simulink model "System_composer__model_pre_alpha_V2"  (R2022b)
settings: Solver=VariableStepAuto  StartTime=0.0  StopTime=10.0  RelTol=1e-3
(part 1 of 3)
settings Model: Creator=user  LastModifiedBy=Sunil Kumar

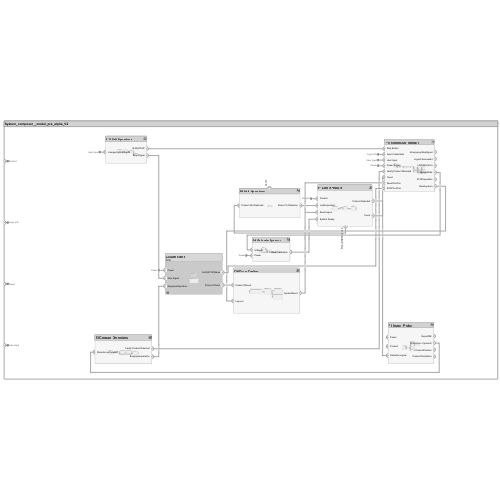
[thumbnail: Simulink's stored preview of the top-level diagram]
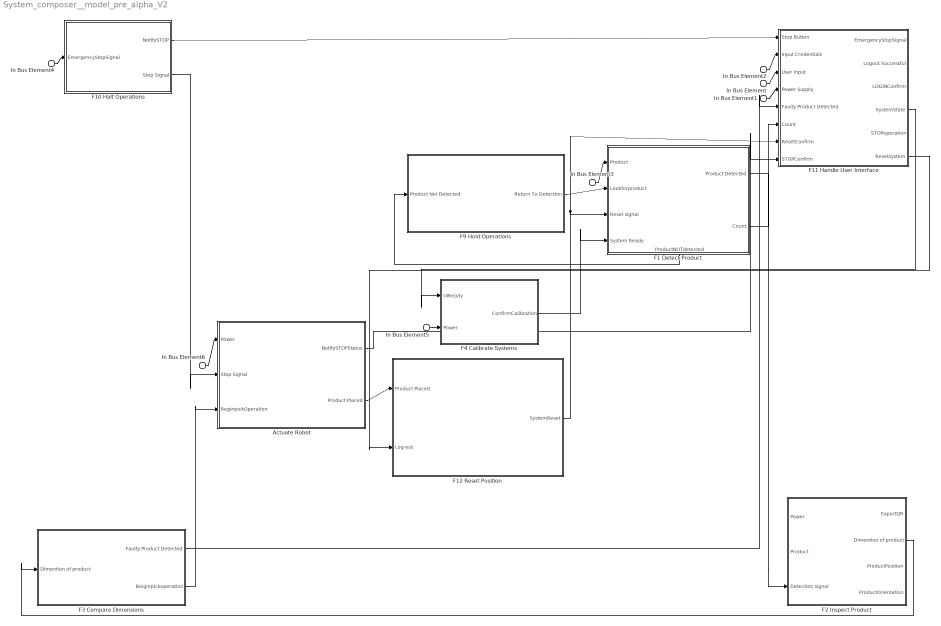
== system System_composer__model_pre_alpha_V2 ==
  In Bus Element3 : Inport  PortName=Product
  In Bus Element2 : Inport  Port=2  PortName=Login info
  In Bus Element1 : Inport  Port=3  PortName=Power
  In Bus Element6 : Inport  Port=3  PortName=Power
  In Bus Element5 : Inport  Port=3  PortName=Power
  In Bus Element : Inport  Port=4  PortName=User Input
  In Bus Element4 : Inport  Port=4  PortName=User Input
  Actuate Robot : Subsystem  Variant=on  VariantControlMode=label  LabelModeActiveChoice=false
      settings: PortSchema="{\"entries\":[{\"content\":{\"headerSize\":38,\"margin\":15,\"minimumSpacing\":25,\"sides\":[{\"content\":{\"connectorIds\":[\"In1\",\"In2\",\"In3\"]},\"type\":\"ConnectorPlacement.EquallySpacedRectSide\",\"uuid\":\"801652fd-f6d1-4274-af0e-cb86f9305aea\"},{\"content\":{\"connectorIds\":[\"Out1\",\"Out2\"],\"side\":\"RIGHT\"},\"type\":\"ConnectorPlacement.EquallySpacedRectSide\",\"uuid\":\"95203280-2c96-4067-b57a-d6395a07757b\"},{\"content\":{\"connectorIds\":[],\"side\":\"TOP\"},\"type\":\"ConnectorPlacement.EquallySpacedRectSide\",\"uuid\":\"56d65509-64de-4fc3-ae90-5c873f468874\"}]},\"type\":\"ConnectorPlacement.EquallySpacedConnector\",\"uuid\":\"1a0d29b8-31f4-46a4-bc3c-cb1d4cb15c15\"}],\"packageUris\":[\"http://schema.mathworks.com/mf0/Connector/R2020b\"],\"version\":\"1.0\"}"
  F1 Detect Product : Subsystem
      settings: PortSchema="{\"entries\":[{\"content\":{\"headerSize\":26,\"margin\":15,\"minimumSpacing\":25,\"sides\":[{\"content\":{\"connectorIds\":[\"In1\",\"In2\",\"In3\",\"In4\"]},\"type\":\"ConnectorPlacement.EquallySpacedRectSide\",\"uuid\":\"0eb90d47-70e1-4803-9acf-c665eca2c33b\"},{\"content\":{\"connectorIds\":[\"Out2\",\"Out3\"],\"side\":\"RIGHT\"},\"type\":\"ConnectorPlacement.EquallySpacedRectSide\",\"uuid\":\"4ca2a7b5-05ae-49c5-bdeb-54cebcfbfa14\"},{\"content\":{\"connectorIds\":[],\"side\":\"TOP\"},\"type\":\"ConnectorPlacement.EquallySpacedRectSide\",\"uuid\":\"0ca0afdf-f9df-4611-9068-250b443486a2\"},{\"content\":{\"connectorIds\":[\"Out1\"],\"side\":\"BOTTOM\"},\"type\":\"ConnectorPlacement.EquallySpacedRectSide\",\"uuid\":\"bd2a3fb3-3c9c-4a9d-a87c-821984a35fa0\"}]},\"type\":\"ConnectorPlacement.EquallySpacedConnector\",\"uuid\":\"958f48af-2ef9-4d0f-b00d-a4686f354a93\"}],\"packageUris\":[\"http://schema.mathworks.com/mf0/Connector/R2020b\"],\"version\":\"1.0\"}"
  F10 Halt Operations : Subsystem
      settings: PortSchema="{\"entries\":[{\"content\":{\"headerSize\":26,\"margin\":15,\"minimumSpacing\":25,\"sides\":[{\"content\":{\"connectorIds\":[\"In1\"]},\"type\":\"ConnectorPlacement.EquallySpacedRectSide\",\"uuid\":\"0eb90d47-70e1-4803-9acf-c665eca2c33b\"},{\"content\":{\"connectorIds\":[\"Out1\",\"Out2\"],\"side\":\"RIGHT\"},\"type\":\"ConnectorPlacement.EquallySpacedRectSide\",\"uuid\":\"4ca2a7b5-05ae-49c5-bdeb-54cebcfbfa14\"},{\"content\":{\"connectorIds\":[],\"side\":\"TOP\"},\"type\":\"ConnectorPlacement.EquallySpacedRectSide\",\"uuid\":\"0ca0afdf-f9df-4611-9068-250b443486a2\"}]},\"type\":\"ConnectorPlacement.EquallySpacedConnector\",\"uuid\":\"958f48af-2ef9-4d0f-b00d-a4686f354a93\"}],\"packageUris\":[\"http://schema.mathworks.com/mf0/Connector/R2020b\"],\"version\":\"1.0\"}"
  F11 Handle User Interface : Subsystem
      settings: PortSchema="{\"entries\":[{\"content\":{\"headerSize\":26,\"margin\":15,\"minimumSpacing\":25,\"sides\":[{\"content\":{\"connectorIds\":[\"In1\",\"In2\",\"In3\",\"In4\",\"In5\",\"In6\",\"In7\",\"In8\"]},\"type\":\"ConnectorPlacement.EquallySpacedRectSide\",\"uuid\":\"0eb90d47-70e1-4803-9acf-c665eca2c33b\"},{\"content\":{\"connectorIds\":[\"Out1\",\"Out2\",\"Out3\",\"Out5\",\"Out6\",\"Out4\"],\"side\":\"RIGHT\"},\"type\":\"ConnectorPlacement.EquallySpacedRectSide\",\"uuid\":\"4ca2a7b5-05ae-49c5-bdeb-54cebcfbfa14\"},{\"content\":{\"connectorIds\":[],\"side\":\"TOP\"},\"type\":\"ConnectorPlacement.EquallySpacedRectSide\",\"uuid\":\"0ca0afdf-f9df-4611-9068-250b443486a2\"}]},\"type\":\"ConnectorPlacement.EquallySpacedConnector\",\"uuid\":\"958f48af-2ef9-4d0f-b00d-a4686f354a93\"}],\"packageUris\":[\"http://schema.mathworks.com/mf0/Connector/R2020b\"],\"version\":\"1.0\"}"
  F12 Reset Position : Subsystem
      settings: PortSchema="{\"entries\":[{\"content\":{\"headerSize\":26,\"margin\":15,\"minimumSpacing\":25,\"sides\":[{\"content\":{\"connectorIds\":[\"In1\",\"In2\"]},\"type\":\"ConnectorPlacement.EquallySpacedRectSide\",\"uuid\":\"1c117138-a6d4-4ec0-b7b8-6d1428745998\"},{\"content\":{\"connectorIds\":[\"Out1\"],\"side\":\"RIGHT\"},\"type\":\"ConnectorPlacement.EquallySpacedRectSide\",\"uuid\":\"426d6ceb-18a6-42d8-9bd7-8fe69cb751f0\"},{\"content\":{\"connectorIds\":[],\"side\":\"TOP\"},\"type\":\"ConnectorPlacement.EquallySpacedRectSide\",\"uuid\":\"23012487-78cd-45b9-9306-44393710ac2e\"}]},\"type\":\"ConnectorPlacement.EquallySpacedConnector\",\"uuid\":\"f4468a7a-13e2-43af-b621-864ee5d109de\"}],\"packageUris\":[\"http://schema.mathworks.com/mf0/Connector/R2020b\"],\"version\":\"1.0\"}"
  F2 Inspect Product : Subsystem
      settings: PortSchema="{\"entries\":[{\"content\":{\"headerSize\":26,\"margin\":15,\"minimumSpacing\":25,\"sides\":[{\"content\":{\"connectorIds\":[\"In1\",\"In2\",\"In3\"]},\"type\":\"ConnectorPlacement.EquallySpacedRectSide\",\"uuid\":\"0eb90d47-70e1-4803-9acf-c665eca2c33b\"},{\"content\":{\"connectorIds\":[\"Out1\",\"Out2\",\"Out3\",\"Out4\"],\"side\":\"RIGHT\"},\"type\":\"ConnectorPlacement.EquallySpacedRectSide\",\"uuid\":\"4ca2a7b5-05ae-49c5-bdeb-54cebcfbfa14\"},{\"content\":{\"connectorIds\":[],\"side\":\"TOP\"},\"type\":\"ConnectorPlacement.EquallySpacedRectSide\",\"uuid\":\"0ca0afdf-f9df-4611-9068-250b443486a2\"}]},\"type\":\"ConnectorPlacement.EquallySpacedConnector\",\"uuid\":\"958f48af-2ef9-4d0f-b00d-a4686f354a93\"}],\"packageUris\":[\"http://schema.mathworks.com/mf0/Connector/R2020b\"],\"version\":\"1.0\"}"
  F3 Compare Dimensions : Subsystem
      settings: PortSchema="{\"entries\":[{\"content\":{\"headerSize\":26,\"margin\":15,\"minimumSpacing\":25,\"sides\":[{\"content\":{\"connectorIds\":[\"In1\"]},\"type\":\"ConnectorPlacement.EquallySpacedRectSide\",\"uuid\":\"0eb90d47-70e1-4803-9acf-c665eca2c33b\"},{\"content\":{\"connectorIds\":[\"Out1\",\"Out2\"],\"side\":\"RIGHT\"},\"type\":\"ConnectorPlacement.EquallySpacedRectSide\",\"uuid\":\"4ca2a7b5-05ae-49c5-bdeb-54cebcfbfa14\"},{\"content\":{\"connectorIds\":[],\"side\":\"TOP\"},\"type\":\"ConnectorPlacement.EquallySpacedRectSide\",\"uuid\":\"0ca0afdf-f9df-4611-9068-250b443486a2\"}]},\"type\":\"ConnectorPlacement.EquallySpacedConnector\",\"uuid\":\"958f48af-2ef9-4d0f-b00d-a4686f354a93\"}],\"packageUris\":[\"http://schema.mathworks.com/mf0/Connector/R2020b\"],\"version\":\"1.0\"}"
  "F4 Calibrate Systems " : Subsystem
      settings: PortSchema="{\"entries\":[{\"content\":{\"headerSize\":26,\"margin\":15,\"minimumSpacing\":25,\"sides\":[{\"content\":{\"connectorIds\":[\"In1\",\"In2\"]},\"type\":\"ConnectorPlacement.EquallySpacedRectSide\",\"uuid\":\"0eb90d47-70e1-4803-9acf-c665eca2c33b\"},{\"content\":{\"connectorIds\":[\"Out1\"],\"side\":\"RIGHT\"},\"type\":\"ConnectorPlacement.EquallySpacedRectSide\",\"uuid\":\"4ca2a7b5-05ae-49c5-bdeb-54cebcfbfa14\"},{\"content\":{\"connectorIds\":[],\"side\":\"TOP\"},\"type\":\"ConnectorPlacement.EquallySpacedRectSide\",\"uuid\":\"0ca0afdf-f9df-4611-9068-250b443486a2\"}]},\"type\":\"ConnectorPlacement.EquallySpacedConnector\",\"uuid\":\"958f48af-2ef9-4d0f-b00d-a4686f354a93\"}],\"packageUris\":[\"http://schema.mathworks.com/mf0/Connector/R2020b\"],\"version\":\"1.0\"}"
  F9 Hold Operations : Subsystem
      settings: PortSchema="{\"entries\":[{\"content\":{\"headerSize\":26,\"margin\":15,\"minimumSpacing\":25,\"sides\":[{\"content\":{\"connectorIds\":[\"In1\"]},\"type\":\"ConnectorPlacement.EquallySpacedRectSide\",\"uuid\":\"0eb90d47-70e1-4803-9acf-c665eca2c33b\"},{\"content\":{\"connectorIds\":[\"Out1\"],\"side\":\"RIGHT\"},\"type\":\"ConnectorPlacement.EquallySpacedRectSide\",\"uuid\":\"4ca2a7b5-05ae-49c5-bdeb-54cebcfbfa14\"},{\"content\":{\"connectorIds\":[\"LConn1\"],\"side\":\"TOP\"},\"type\":\"ConnectorPlacement.EquallySpacedRectSide\",\"uuid\":\"0ca0afdf-f9df-4611-9068-250b443486a2\"}]},\"type\":\"ConnectorPlacement.EquallySpacedConnector\",\"uuid\":\"958f48af-2ef9-4d0f-b00d-a4686f354a93\"}],\"packageUris\":[\"http://schema.mathworks.com/mf0/Connector/R2020b\"],\"version\":\"1.0\"}"
  wires:
  In Bus Element4/1 -> F10 Halt Operations/1(EmergencyStopSignal)
  F10 Halt Operations/1(NotifySTOP) -> F11 Handle User Interface/1(Stop Button)
  F3 Compare Dimensions/2(Beiginpickoperation) -> Actuate Robot/3(BeginpickOperation)
  F3 Compare Dimensions/1(Faulty Product Detected) -> F11 Handle User Interface/5(Faulty Product Detected)
  F1 Detect Product/2(Product Detected) -> F2 Inspect Product/3(Detection signal)
  F10 Halt Operations/2(Stop Signal) -> Actuate Robot/2(Stop Signal)
  Actuate Robot/2(Product Placed) -> F12 Reset Position/1(Product Placed)
  In Bus Element6/1 -> Actuate Robot/1(Power)
  F11 Handle User Interface/4(Resetsystem) -> F12 Reset Position/2(Log-out)
  Actuate Robot/1(NotifySTOPStatus) -> F11 Handle User Interface/8(STOPConfirm)
  In Bus Element5/1 -> "F4 Calibrate Systems "/2(Power)
  In Bus Element3/1 -> F1 Detect Product/1(Product)
  F9 Hold Operations/1(Return To Detection) -> F1 Detect Product/2(Lookforproduct)
  "F4 Calibrate Systems "/1(ConfirmCalibration) -> F1 Detect Product/4(System Ready)
  F12 Reset Position/1(SystemReset) -> F11 Handle User Interface/7(ResetConfirm), F1 Detect Product/3(Reset signal)
  F1 Detect Product/3(Count) -> F11 Handle User Interface/6(Count)
  F1 Detect Product/1(ProductNOTdetected) -> F9 Hold Operations/1(Product Not Detected)
  In Bus Element2/1 -> F11 Handle User Interface/2(Input Credentials)
  In Bus Element/1 -> F11 Handle User Interface/3(User Input)
  In Bus Element1/1 -> F11 Handle User Interface/4(Power Supply)
  F11 Handle User Interface/5(SystemState) -> "F4 Calibrate Systems "/1(UIReady)
  F2 Inspect Product/2(Dimention of product) -> F3 Compare Dimensions/1(Dimention of product)

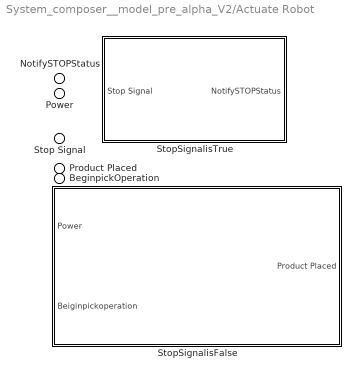
== system System_composer__model_pre_alpha_V2/Actuate Robot ==
  Power : Inport
  Stop Signal : Inport  Port=2
  BeginpickOperation : Inport  Port=3
  StopSignalisFalse : Subsystem  VariantControl=false
      settings: PortSchema="{\"entries\":[{\"content\":{\"headerSize\":26,\"margin\":15,\"minimumSpacing\":25,\"sides\":[{\"content\":{\"connectorIds\":[\"In1\",\"In2\"]},\"type\":\"ConnectorPlacement.EquallySpacedRectSide\",\"uuid\":\"48af5bc1-3520-4798-93f0-e999f4a2b359\"},{\"content\":{\"connectorIds\":[\"Out1\"],\"side\":\"RIGHT\"},\"type\":\"ConnectorPlacement.EquallySpacedRectSide\",\"uuid\":\"b080505c-f688-49a6-aa0b-291a70fb9613\"},{\"content\":{\"connectorIds\":[],\"side\":\"TOP\"},\"type\":\"ConnectorPlacement.EquallySpacedRectSide\",\"uuid\":\"3b22725c-7b13-4de8-bd12-2bd6e95657e0\"}]},\"type\":\"ConnectorPlacement.EquallySpacedConnector\",\"uuid\":\"97afaf3e-8205-465e-91b8-6c9d28738099\"}],\"packageUris\":[\"http://schema.mathworks.com/mf0/Connector/R2020b\"],\"version\":\"1.0\"}"
  StopSignalisTrue : Subsystem  VariantControl=true
      settings: PortSchema="{\"entries\":[{\"content\":{\"headerSize\":26,\"margin\":15,\"minimumSpacing\":25,\"sides\":[{\"content\":{\"connectorIds\":[\"In1\"]},\"type\":\"ConnectorPlacement.EquallySpacedRectSide\",\"uuid\":\"48af5bc1-3520-4798-93f0-e999f4a2b359\"},{\"content\":{\"connectorIds\":[\"Out1\"],\"side\":\"RIGHT\"},\"type\":\"ConnectorPlacement.EquallySpacedRectSide\",\"uuid\":\"b080505c-f688-49a6-aa0b-291a70fb9613\"},{\"content\":{\"connectorIds\":[],\"side\":\"TOP\"},\"type\":\"ConnectorPlacement.EquallySpacedRectSide\",\"uuid\":\"3b22725c-7b13-4de8-bd12-2bd6e95657e0\"}]},\"type\":\"ConnectorPlacement.EquallySpacedConnector\",\"uuid\":\"97afaf3e-8205-465e-91b8-6c9d28738099\"}],\"packageUris\":[\"http://schema.mathworks.com/mf0/Connector/R2020b\"],\"version\":\"1.0\"}"
  NotifySTOPStatus : Outport
  Product Placed : Outport  Port=2

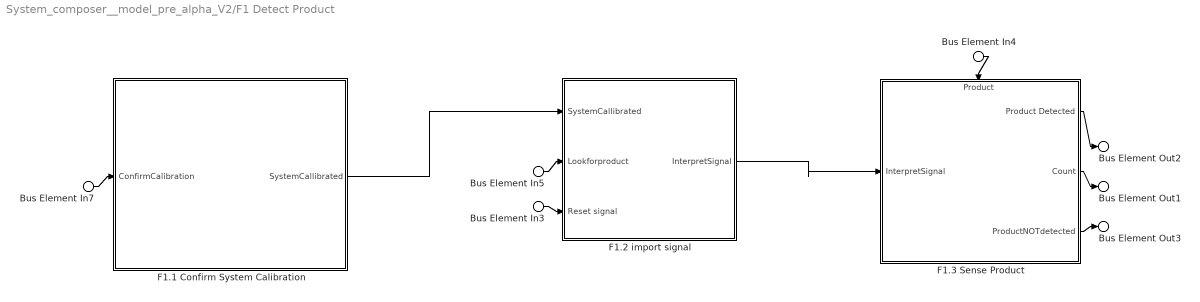
== system System_composer__model_pre_alpha_V2/F1 Detect Product ==
  Bus Element In4 : Inport  PortName=Product
  Bus Element In5 : Inport  Port=2  PortName=Lookforproduct
  Bus Element In3 : Inport  Port=3  PortName=Reset signal
  Bus Element In7 : Inport  Port=4  PortName=System Ready
  F1.1 Confirm System Calibration : Subsystem
      settings: PortSchema="{\"entries\":[{\"content\":{\"headerSize\":26,\"margin\":15,\"minimumSpacing\":25,\"sides\":[{\"content\":{\"connectorIds\":[\"In1\"]},\"type\":\"ConnectorPlacement.EquallySpacedRectSide\",\"uuid\":\"ae240f5f-39ed-41a3-b9a8-bf2f33b986be\"},{\"content\":{\"connectorIds\":[\"Out1\"],\"side\":\"RIGHT\"},\"type\":\"ConnectorPlacement.EquallySpacedRectSide\",\"uuid\":\"44ba199a-fd12-4621-8565-f3f1adedec4a\"},{\"content\":{\"connectorIds\":[],\"side\":\"TOP\"},\"type\":\"ConnectorPlacement.EquallySpacedRectSide\",\"uuid\":\"41d301d8-0f91-4ed1-b07b-750dd04e1ae2\"}]},\"type\":\"ConnectorPlacement.EquallySpacedConnector\",\"uuid\":\"8d081691-644b-416f-87ea-d7e0a52b2ce6\"}],\"packageUris\":[\"http://schema.mathworks.com/mf0/Connector/R2020b\"],\"version\":\"1.0\"}"
  F1.2 import signal : Subsystem
      settings: PortSchema="{\"entries\":[{\"content\":{\"headerSize\":26,\"margin\":15,\"minimumSpacing\":25,\"sides\":[{\"content\":{\"connectorIds\":[\"In1\",\"In2\",\"In3\"]},\"type\":\"ConnectorPlacement.EquallySpacedRectSide\",\"uuid\":\"ee97644e-c9ff-4946-8a58-fee1d557a4ad\"},{\"content\":{\"connectorIds\":[\"Out1\"],\"side\":\"RIGHT\"},\"type\":\"ConnectorPlacement.EquallySpacedRectSide\",\"uuid\":\"e20fd496-d0ba-45f7-949d-94f28912a261\"},{\"content\":{\"connectorIds\":[],\"side\":\"TOP\"},\"type\":\"ConnectorPlacement.EquallySpacedRectSide\",\"uuid\":\"6224eb33-55c0-4770-9979-a18202099dbf\"}]},\"type\":\"ConnectorPlacement.EquallySpacedConnector\",\"uuid\":\"f8ef62f6-ad53-4f25-bdc3-ef7ca131dedb\"}],\"packageUris\":[\"http://schema.mathworks.com/mf0/Connector/R2020b\"],\"version\":\"1.0\"}"
  F1.3 Sense Product : Subsystem
      settings: PortSchema="{\"entries\":[{\"content\":{\"headerSize\":26,\"margin\":15,\"minimumSpacing\":25,\"sides\":[{\"content\":{\"connectorIds\":[\"In2\"]},\"type\":\"ConnectorPlacement.EquallySpacedRectSide\",\"uuid\":\"ee97644e-c9ff-4946-8a58-fee1d557a4ad\"},{\"content\":{\"connectorIds\":[\"Out1\",\"Out2\",\"Out3\"],\"side\":\"RIGHT\"},\"type\":\"ConnectorPlacement.EquallySpacedRectSide\",\"uuid\":\"e20fd496-d0ba-45f7-949d-94f28912a261\"},{\"content\":{\"connectorIds\":[\"In1\"],\"side\":\"TOP\"},\"type\":\"ConnectorPlacement.EquallySpacedRectSide\",\"uuid\":\"6224eb33-55c0-4770-9979-a18202099dbf\"}]},\"type\":\"ConnectorPlacement.EquallySpacedConnector\",\"uuid\":\"f8ef62f6-ad53-4f25-bdc3-ef7ca131dedb\"}],\"packageUris\":[\"http://schema.mathworks.com/mf0/Connector/R2020b\"],\"version\":\"1.0\"}"
  Bus Element Out3 : Outport  PortName=ProductNOTdetected
  Bus Element Out2 : Outport  Port=2  PortName=Product Detected
  Bus Element Out1 : Outport  Port=3  PortName=Count
  wires:
  Bus Element In3/1 -> F1.2 import signal/3(Reset signal)
  F1.2 import signal/1(InterpretSignal) -> F1.3 Sense Product/2(InterpretSignal)
  Bus Element In4/1 -> F1.3 Sense Product/1(Product)
  F1.3 Sense Product/2(Count) -> Bus Element Out1/1
  F1.3 Sense Product/1(Product Detected) -> Bus Element Out2/1
  F1.3 Sense Product/3(ProductNOTdetected) -> Bus Element Out3/1
  Bus Element In5/1 -> F1.2 import signal/2(Lookforproduct)
  F1.1 Confirm System Calibration/1(SystemCallibrated) -> F1.2 import signal/1(SystemCallibrated)
  Bus Element In7/1 -> F1.1 Confirm System Calibration/1(ConfirmCalibration)

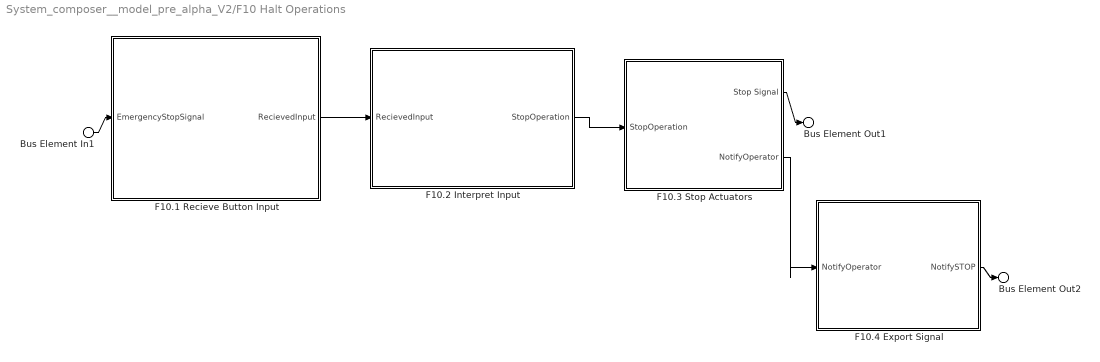
== system System_composer__model_pre_alpha_V2/F10 Halt Operations ==
  Bus Element In1 : Inport  PortName=EmergencyStopSignal
  F10.1 Recieve Button Input : Subsystem
      settings: PortSchema="{\"entries\":[{\"content\":{\"headerSize\":26,\"margin\":15,\"minimumSpacing\":25,\"sides\":[{\"content\":{\"connectorIds\":[\"In1\"]},\"type\":\"ConnectorPlacement.EquallySpacedRectSide\",\"uuid\":\"7013333b-bcb0-472a-8b4b-201a684e0f69\"},{\"content\":{\"connectorIds\":[\"Out1\"],\"side\":\"RIGHT\"},\"type\":\"ConnectorPlacement.EquallySpacedRectSide\",\"uuid\":\"4b4cc890-b976-4837-92a8-5b6c4ad3f659\"},{\"content\":{\"connectorIds\":[],\"side\":\"TOP\"},\"type\":\"ConnectorPlacement.EquallySpacedRectSide\",\"uuid\":\"d943cfaa-ae22-4a3b-a19a-c6fb5e90d8f6\"}]},\"type\":\"ConnectorPlacement.EquallySpacedConnector\",\"uuid\":\"02e5c76f-f132-4257-84b4-ea3020272a7a\"}],\"packageUris\":[\"http://schema.mathworks.com/mf0/Connector/R2020b\"],\"version\":\"1.0\"}"
  F10.2 Interpret Input : Subsystem
      settings: PortSchema="{\"entries\":[{\"content\":{\"headerSize\":26,\"margin\":15,\"minimumSpacing\":25,\"sides\":[{\"content\":{\"connectorIds\":[\"In1\"]},\"type\":\"ConnectorPlacement.EquallySpacedRectSide\",\"uuid\":\"7013333b-bcb0-472a-8b4b-201a684e0f69\"},{\"content\":{\"connectorIds\":[\"Out1\"],\"side\":\"RIGHT\"},\"type\":\"ConnectorPlacement.EquallySpacedRectSide\",\"uuid\":\"4b4cc890-b976-4837-92a8-5b6c4ad3f659\"},{\"content\":{\"connectorIds\":[],\"side\":\"TOP\"},\"type\":\"ConnectorPlacement.EquallySpacedRectSide\",\"uuid\":\"d943cfaa-ae22-4a3b-a19a-c6fb5e90d8f6\"}]},\"type\":\"ConnectorPlacement.EquallySpacedConnector\",\"uuid\":\"02e5c76f-f132-4257-84b4-ea3020272a7a\"}],\"packageUris\":[\"http://schema.mathworks.com/mf0/Connector/R2020b\"],\"version\":\"1.0\"}"
  F10.3 Stop Actuators : Subsystem
      settings: PortSchema="{\"entries\":[{\"content\":{\"headerSize\":26,\"margin\":15,\"minimumSpacing\":25,\"sides\":[{\"content\":{\"connectorIds\":[\"In1\"]},\"type\":\"ConnectorPlacement.EquallySpacedRectSide\",\"uuid\":\"7013333b-bcb0-472a-8b4b-201a684e0f69\"},{\"content\":{\"connectorIds\":[\"Out2\",\"Out1\"],\"side\":\"RIGHT\"},\"type\":\"ConnectorPlacement.EquallySpacedRectSide\",\"uuid\":\"4b4cc890-b976-4837-92a8-5b6c4ad3f659\"},{\"content\":{\"connectorIds\":[],\"side\":\"TOP\"},\"type\":\"ConnectorPlacement.EquallySpacedRectSide\",\"uuid\":\"d943cfaa-ae22-4a3b-a19a-c6fb5e90d8f6\"}]},\"type\":\"ConnectorPlacement.EquallySpacedConnector\",\"uuid\":\"02e5c76f-f132-4257-84b4-ea3020272a7a\"}],\"packageUris\":[\"http://schema.mathworks.com/mf0/Connector/R2020b\"],\"version\":\"1.0\"}"
  F10.4 Export Signal : Subsystem
      settings: PortSchema="{\"entries\":[{\"content\":{\"headerSize\":26,\"margin\":15,\"minimumSpacing\":25,\"sides\":[{\"content\":{\"connectorIds\":[\"In1\"]},\"type\":\"ConnectorPlacement.EquallySpacedRectSide\",\"uuid\":\"7013333b-bcb0-472a-8b4b-201a684e0f69\"},{\"content\":{\"connectorIds\":[\"Out1\"],\"side\":\"RIGHT\"},\"type\":\"ConnectorPlacement.EquallySpacedRectSide\",\"uuid\":\"4b4cc890-b976-4837-92a8-5b6c4ad3f659\"},{\"content\":{\"connectorIds\":[],\"side\":\"TOP\"},\"type\":\"ConnectorPlacement.EquallySpacedRectSide\",\"uuid\":\"d943cfaa-ae22-4a3b-a19a-c6fb5e90d8f6\"}]},\"type\":\"ConnectorPlacement.EquallySpacedConnector\",\"uuid\":\"02e5c76f-f132-4257-84b4-ea3020272a7a\"}],\"packageUris\":[\"http://schema.mathworks.com/mf0/Connector/R2020b\"],\"version\":\"1.0\"}"
  Bus Element Out2 : Outport  PortName=NotifySTOP
  Bus Element Out1 : Outport  Port=2  PortName=Stop Signal
  wires:
  F10.3 Stop Actuators/2(Stop Signal) -> Bus Element Out1/1
  Bus Element In1/1 -> F10.1 Recieve Button Input/1(EmergencyStopSignal)
  F10.1 Recieve Button Input/1(RecievedInput) -> F10.2 Interpret Input/1(RecievedInput)
  F10.2 Interpret Input/1(StopOperation) -> F10.3 Stop Actuators/1(StopOperation)
  F10.3 Stop Actuators/1(NotifyOperator) -> F10.4 Export Signal/1(NotifyOperator)
  F10.4 Export Signal/1(NotifySTOP) -> Bus Element Out2/1

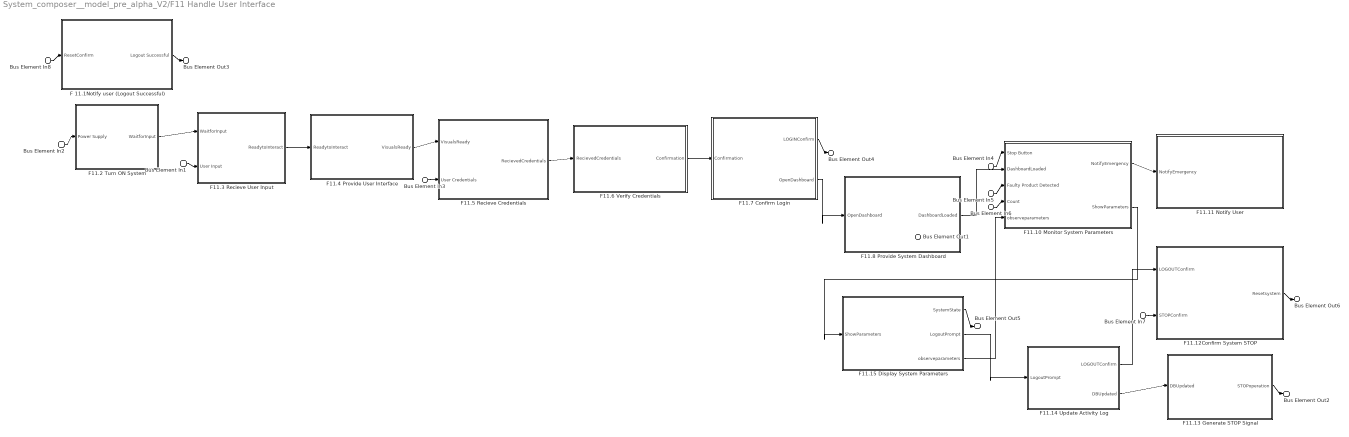
== system System_composer__model_pre_alpha_V2/F11 Handle User Interface ==
  Bus Element In4 : Inport  PortName=Stop Button
  Bus Element In3 : Inport  Port=2  PortName=Input Credentials
  Bus Element In1 : Inport  Port=3  PortName=User Input
  Bus Element In2 : Inport  Port=4  PortName=Power Supply
  Bus Element In5 : Inport  Port=5  PortName=Faulty Product Detected
  Bus Element In6 : Inport  Port=6  PortName=Count
  Bus Element In8 : Inport  Port=7  PortName=ResetConfirm
  Bus Element In7 : Inport  Port=8  PortName=STOPConfirm
  F 11.1Notify user (Logout Successful) : Subsystem
      settings: PortSchema="{\"entries\":[{\"content\":{\"headerSize\":26,\"margin\":15,\"minimumSpacing\":25,\"sides\":[{\"content\":{\"connectorIds\":[\"In1\"]},\"type\":\"ConnectorPlacement.EquallySpacedRectSide\",\"uuid\":\"ae240f5f-39ed-41a3-b9a8-bf2f33b986be\"},{\"content\":{\"connectorIds\":[\"Out1\"],\"side\":\"RIGHT\"},\"type\":\"ConnectorPlacement.EquallySpacedRectSide\",\"uuid\":\"44ba199a-fd12-4621-8565-f3f1adedec4a\"},{\"content\":{\"connectorIds\":[],\"side\":\"TOP\"},\"type\":\"ConnectorPlacement.EquallySpacedRectSide\",\"uuid\":\"41d301d8-0f91-4ed1-b07b-750dd04e1ae2\"}]},\"type\":\"ConnectorPlacement.EquallySpacedConnector\",\"uuid\":\"8d081691-644b-416f-87ea-d7e0a52b2ce6\"}],\"packageUris\":[\"http://schema.mathworks.com/mf0/Connector/R2020b\"],\"version\":\"1.0\"}"
  F11.10 Monitor System Parameters : Subsystem
      settings: PortSchema="{\"entries\":[{\"content\":{\"headerSize\":26,\"margin\":15,\"minimumSpacing\":25,\"sides\":[{\"content\":{\"connectorIds\":[\"In1\",\"In2\",\"In3\",\"In5\",\"In4\"]},\"type\":\"ConnectorPlacement.EquallySpacedRectSide\",\"uuid\":\"0eb90d47-70e1-4803-9acf-c665eca2c33b\"},{\"content\":{\"connectorIds\":[\"Out1\",\"Out2\"],\"side\":\"RIGHT\"},\"type\":\"ConnectorPlacement.EquallySpacedRectSide\",\"uuid\":\"4ca2a7b5-05ae-49c5-bdeb-54cebcfbfa14\"},{\"content\":{\"connectorIds\":[],\"side\":\"TOP\"},\"type\":\"ConnectorPlacement.EquallySpacedRectSide\",\"uuid\":\"0ca0afdf-f9df-4611-9068-250b443486a2\"}]},\"type\":\"ConnectorPlacement.EquallySpacedConnector\",\"uuid\":\"958f48af-2ef9-4d0f-b00d-a4686f354a93\"}],\"packageUris\":[\"http://schema.mathworks.com/mf0/Connector/R2020b\"],\"version\":\"1.0\"}"
  F11.11 Notify User : Subsystem
      settings: PortSchema="{\"entries\":[{\"content\":{\"headerSize\":26,\"margin\":15,\"minimumSpacing\":25,\"sides\":[{\"content\":{\"connectorIds\":[\"In1\"]},\"type\":\"ConnectorPlacement.EquallySpacedRectSide\",\"uuid\":\"0eb90d47-70e1-4803-9acf-c665eca2c33b\"},{\"content\":{\"connectorIds\":[],\"side\":\"RIGHT\"},\"type\":\"ConnectorPlacement.EquallySpacedRectSide\",\"uuid\":\"4ca2a7b5-05ae-49c5-bdeb-54cebcfbfa14\"},{\"content\":{\"connectorIds\":[],\"side\":\"TOP\"},\"type\":\"ConnectorPlacement.EquallySpacedRectSide\",\"uuid\":\"0ca0afdf-f9df-4611-9068-250b443486a2\"}]},\"type\":\"ConnectorPlacement.EquallySpacedConnector\",\"uuid\":\"958f48af-2ef9-4d0f-b00d-a4686f354a93\"}],\"packageUris\":[\"http://schema.mathworks.com/mf0/Connector/R2020b\"],\"version\":\"1.0\"}"
  F11.12Confirm System STOP : Subsystem
      settings: PortSchema="{\"entries\":[{\"content\":{\"headerSize\":26,\"margin\":15,\"minimumSpacing\":25,\"sides\":[{\"content\":{\"connectorIds\":[\"In1\",\"In2\"]},\"type\":\"ConnectorPlacement.EquallySpacedRectSide\",\"uuid\":\"ae240f5f-39ed-41a3-b9a8-bf2f33b986be\"},{\"content\":{\"connectorIds\":[\"Out1\"],\"side\":\"RIGHT\"},\"type\":\"ConnectorPlacement.EquallySpacedRectSide\",\"uuid\":\"44ba199a-fd12-4621-8565-f3f1adedec4a\"},{\"content\":{\"connectorIds\":[],\"side\":\"TOP\"},\"type\":\"ConnectorPlacement.EquallySpacedRectSide\",\"uuid\":\"41d301d8-0f91-4ed1-b07b-750dd04e1ae2\"}]},\"type\":\"ConnectorPlacement.EquallySpacedConnector\",\"uuid\":\"8d081691-644b-416f-87ea-d7e0a52b2ce6\"}],\"packageUris\":[\"http://schema.mathworks.com/mf0/Connector/R2020b\"],\"version\":\"1.0\"}"
  F11.13 Generate STOP Signal : Subsystem
      settings: PortSchema="{\"entries\":[{\"content\":{\"headerSize\":26,\"margin\":15,\"minimumSpacing\":25,\"sides\":[{\"content\":{\"connectorIds\":[\"In1\"]},\"type\":\"ConnectorPlacement.EquallySpacedRectSide\",\"uuid\":\"0eb90d47-70e1-4803-9acf-c665eca2c33b\"},{\"content\":{\"connectorIds\":[\"Out1\"],\"side\":\"RIGHT\"},\"type\":\"ConnectorPlacement.EquallySpacedRectSide\",\"uuid\":\"4ca2a7b5-05ae-49c5-bdeb-54cebcfbfa14\"},{\"content\":{\"connectorIds\":[],\"side\":\"TOP\"},\"type\":\"ConnectorPlacement.EquallySpacedRectSide\",\"uuid\":\"0ca0afdf-f9df-4611-9068-250b443486a2\"}]},\"type\":\"ConnectorPlacement.EquallySpacedConnector\",\"uuid\":\"958f48af-2ef9-4d0f-b00d-a4686f354a93\"}],\"packageUris\":[\"http://schema.mathworks.com/mf0/Connector/R2020b\"],\"version\":\"1.0\"}"
  F11.14 Update Activity Log : Subsystem
      settings: PortSchema="{\"entries\":[{\"content\":{\"headerSize\":26,\"margin\":15,\"minimumSpacing\":25,\"sides\":[{\"content\":{\"connectorIds\":[\"In1\"]},\"type\":\"ConnectorPlacement.EquallySpacedRectSide\",\"uuid\":\"0eb90d47-70e1-4803-9acf-c665eca2c33b\"},{\"content\":{\"connectorIds\":[\"Out1\",\"Out2\"],\"side\":\"RIGHT\"},\"type\":\"ConnectorPlacement.EquallySpacedRectSide\",\"uuid\":\"4ca2a7b5-05ae-49c5-bdeb-54cebcfbfa14\"},{\"content\":{\"connectorIds\":[],\"side\":\"TOP\"},\"type\":\"ConnectorPlacement.EquallySpacedRectSide\",\"uuid\":\"0ca0afdf-f9df-4611-9068-250b443486a2\"}]},\"type\":\"ConnectorPlacement.EquallySpacedConnector\",\"uuid\":\"958f48af-2ef9-4d0f-b00d-a4686f354a93\"}],\"packageUris\":[\"http://schema.mathworks.com/mf0/Connector/R2020b\"],\"version\":\"1.0\"}"
  F11.15 Display System Parameters : Subsystem
      settings: PortSchema="{\"entries\":[{\"content\":{\"headerSize\":26,\"margin\":15,\"minimumSpacing\":25,\"sides\":[{\"content\":{\"connectorIds\":[\"In1\"]},\"type\":\"ConnectorPlacement.EquallySpacedRectSide\",\"uuid\":\"0eb90d47-70e1-4803-9acf-c665eca2c33b\"},{\"content\":{\"connectorIds\":[\"Out1\",\"Out2\",\"Out3\"],\"side\":\"RIGHT\"},\"type\":\"ConnectorPlacement.EquallySpacedRectSide\",\"uuid\":\"4ca2a7b5-05ae-49c5-bdeb-54cebcfbfa14\"},{\"content\":{\"connectorIds\":[],\"side\":\"TOP\"},\"type\":\"ConnectorPlacement.EquallySpacedRectSide\",\"uuid\":\"0ca0afdf-f9df-4611-9068-250b443486a2\"}]},\"type\":\"ConnectorPlacement.EquallySpacedConnector\",\"uuid\":\"958f48af-2ef9-4d0f-b00d-a4686f354a93\"}],\"packageUris\":[\"http://schema.mathworks.com/mf0/Connector/R2020b\"],\"version\":\"1.0\"}"
  F11.2 Turn ON System : Subsystem
      settings: PortSchema="{\"entries\":[{\"content\":{\"headerSize\":26,\"margin\":15,\"minimumSpacing\":25,\"sides\":[{\"content\":{\"connectorIds\":[\"In1\"]},\"type\":\"ConnectorPlacement.EquallySpacedRectSide\",\"uuid\":\"0eb90d47-70e1-4803-9acf-c665eca2c33b\"},{\"content\":{\"connectorIds\":[\"Out1\"],\"side\":\"RIGHT\"},\"type\":\"ConnectorPlacement.EquallySpacedRectSide\",\"uuid\":\"4ca2a7b5-05ae-49c5-bdeb-54cebcfbfa14\"},{\"content\":{\"connectorIds\":[],\"side\":\"TOP\"},\"type\":\"ConnectorPlacement.EquallySpacedRectSide\",\"uuid\":\"0ca0afdf-f9df-4611-9068-250b443486a2\"}]},\"type\":\"ConnectorPlacement.EquallySpacedConnector\",\"uuid\":\"958f48af-2ef9-4d0f-b00d-a4686f354a93\"}],\"packageUris\":[\"http://schema.mathworks.com/mf0/Connector/R2020b\"],\"version\":\"1.0\"}"
  F11.3 Recieve User Input : Subsystem
      settings: PortSchema="{\"entries\":[{\"content\":{\"headerSize\":26,\"margin\":15,\"minimumSpacing\":25,\"sides\":[{\"content\":{\"connectorIds\":[\"In1\",\"In2\"]},\"type\":\"ConnectorPlacement.EquallySpacedRectSide\",\"uuid\":\"0eb90d47-70e1-4803-9acf-c665eca2c33b\"},{\"content\":{\"connectorIds\":[\"Out1\"],\"side\":\"RIGHT\"},\"type\":\"ConnectorPlacement.EquallySpacedRectSide\",\"uuid\":\"4ca2a7b5-05ae-49c5-bdeb-54cebcfbfa14\"},{\"content\":{\"connectorIds\":[],\"side\":\"TOP\"},\"type\":\"ConnectorPlacement.EquallySpacedRectSide\",\"uuid\":\"0ca0afdf-f9df-4611-9068-250b443486a2\"}]},\"type\":\"ConnectorPlacement.EquallySpacedConnector\",\"uuid\":\"958f48af-2ef9-4d0f-b00d-a4686f354a93\"}],\"packageUris\":[\"http://schema.mathworks.com/mf0/Connector/R2020b\"],\"version\":\"1.0\"}"
  F11.4 Provide User Interface : Subsystem
      settings: PortSchema="{\"entries\":[{\"content\":{\"headerSize\":26,\"margin\":15,\"minimumSpacing\":25,\"sides\":[{\"content\":{\"connectorIds\":[\"In1\"]},\"type\":\"ConnectorPlacement.EquallySpacedRectSide\",\"uuid\":\"0eb90d47-70e1-4803-9acf-c665eca2c33b\"},{\"content\":{\"connectorIds\":[\"Out1\"],\"side\":\"RIGHT\"},\"type\":\"ConnectorPlacement.EquallySpacedRectSide\",\"uuid\":\"4ca2a7b5-05ae-49c5-bdeb-54cebcfbfa14\"},{\"content\":{\"connectorIds\":[],\"side\":\"TOP\"},\"type\":\"ConnectorPlacement.EquallySpacedRectSide\",\"uuid\":\"0ca0afdf-f9df-4611-9068-250b443486a2\"}]},\"type\":\"ConnectorPlacement.EquallySpacedConnector\",\"uuid\":\"958f48af-2ef9-4d0f-b00d-a4686f354a93\"}],\"packageUris\":[\"http://schema.mathworks.com/mf0/Connector/R2020b\"],\"version\":\"1.0\"}"
  F11.5 Recieve Credentials : Subsystem
      settings: PortSchema="{\"entries\":[{\"content\":{\"headerSize\":26,\"margin\":15,\"minimumSpacing\":25,\"sides\":[{\"content\":{\"connectorIds\":[\"In1\",\"In2\"]},\"type\":\"ConnectorPlacement.EquallySpacedRectSide\",\"uuid\":\"0eb90d47-70e1-4803-9acf-c665eca2c33b\"},{\"content\":{\"connectorIds\":[\"Out1\"],\"side\":\"RIGHT\"},\"type\":\"ConnectorPlacement.EquallySpacedRectSide\",\"uuid\":\"4ca2a7b5-05ae-49c5-bdeb-54cebcfbfa14\"},{\"content\":{\"connectorIds\":[],\"side\":\"TOP\"},\"type\":\"ConnectorPlacement.EquallySpacedRectSide\",\"uuid\":\"0ca0afdf-f9df-4611-9068-250b443486a2\"}]},\"type\":\"ConnectorPlacement.EquallySpacedConnector\",\"uuid\":\"958f48af-2ef9-4d0f-b00d-a4686f354a93\"}],\"packageUris\":[\"http://schema.mathworks.com/mf0/Connector/R2020b\"],\"version\":\"1.0\"}"
  F11.6 Verify Credentials : Subsystem
      settings: PortSchema="{\"entries\":[{\"content\":{\"headerSize\":26,\"margin\":15,\"minimumSpacing\":25,\"sides\":[{\"content\":{\"connectorIds\":[\"In1\"]},\"type\":\"ConnectorPlacement.EquallySpacedRectSide\",\"uuid\":\"0eb90d47-70e1-4803-9acf-c665eca2c33b\"},{\"content\":{\"connectorIds\":[\"Out1\"],\"side\":\"RIGHT\"},\"type\":\"ConnectorPlacement.EquallySpacedRectSide\",\"uuid\":\"4ca2a7b5-05ae-49c5-bdeb-54cebcfbfa14\"},{\"content\":{\"connectorIds\":[],\"side\":\"TOP\"},\"type\":\"ConnectorPlacement.EquallySpacedRectSide\",\"uuid\":\"0ca0afdf-f9df-4611-9068-250b443486a2\"}]},\"type\":\"ConnectorPlacement.EquallySpacedConnector\",\"uuid\":\"958f48af-2ef9-4d0f-b00d-a4686f354a93\"}],\"packageUris\":[\"http://schema.mathworks.com/mf0/Connector/R2020b\"],\"version\":\"1.0\"}"
  F11.7 Confirm Login : Subsystem
      settings: PortSchema="{\"entries\":[{\"content\":{\"headerSize\":26,\"margin\":15,\"minimumSpacing\":25,\"sides\":[{\"content\":{\"connectorIds\":[\"In1\"]},\"type\":\"ConnectorPlacement.EquallySpacedRectSide\",\"uuid\":\"0eb90d47-70e1-4803-9acf-c665eca2c33b\"},{\"content\":{\"connectorIds\":[\"Out1\",\"Out2\"],\"side\":\"RIGHT\"},\"type\":\"ConnectorPlacement.EquallySpacedRectSide\",\"uuid\":\"4ca2a7b5-05ae-49c5-bdeb-54cebcfbfa14\"},{\"content\":{\"connectorIds\":[],\"side\":\"TOP\"},\"type\":\"ConnectorPlacement.EquallySpacedRectSide\",\"uuid\":\"0ca0afdf-f9df-4611-9068-250b443486a2\"}]},\"type\":\"ConnectorPlacement.EquallySpacedConnector\",\"uuid\":\"958f48af-2ef9-4d0f-b00d-a4686f354a93\"}],\"packageUris\":[\"http://schema.mathworks.com/mf0/Connector/R2020b\"],\"version\":\"1.0\"}"
  F11.8 Provide System Dashboard : Subsystem
      settings: PortSchema="{\"entries\":[{\"content\":{\"headerSize\":26,\"margin\":15,\"minimumSpacing\":25,\"sides\":[{\"content\":{\"connectorIds\":[\"In1\"]},\"type\":\"ConnectorPlacement.EquallySpacedRectSide\",\"uuid\":\"0eb90d47-70e1-4803-9acf-c665eca2c33b\"},{\"content\":{\"connectorIds\":[\"Out1\"],\"side\":\"RIGHT\"},\"type\":\"ConnectorPlacement.EquallySpacedRectSide\",\"uuid\":\"4ca2a7b5-05ae-49c5-bdeb-54cebcfbfa14\"},{\"content\":{\"connectorIds\":[],\"side\":\"TOP\"},\"type\":\"ConnectorPlacement.EquallySpacedRectSide\",\"uuid\":\"0ca0afdf-f9df-4611-9068-250b443486a2\"}]},\"type\":\"ConnectorPlacement.EquallySpacedConnector\",\"uuid\":\"958f48af-2ef9-4d0f-b00d-a4686f354a93\"}],\"packageUris\":[\"http://schema.mathworks.com/mf0/Connector/R2020b\"],\"version\":\"1.0\"}"
  Bus Element Out1 : Outport  PortName=EmergencyStopSignal
  Bus Element Out3 : Outport  Port=2  PortName=Logout Successful
  Bus Element Out4 : Outport  Port=3  PortName=LOGINConfirm
  Bus Element Out6 : Outport  Port=4  PortName=Resetsystem
  Bus Element Out5 : Outport  Port=5  PortName=SystemState
  Bus Element Out2 : Outport  Port=6  PortName=STOPoperation
  wires:
  Bus Element In3/1 -> F11.5 Recieve Credentials/2(User Credentials)
  F11.7 Confirm Login/2(OpenDashboard) -> F11.8 Provide System Dashboard/1(OpenDashboard)
  Bus Element In1/1 -> F11.3 Recieve User Input/2(User Input)
  Bus Element In2/1 -> F11.2 Turn ON System/1(Power Supply)
  Bus Element In8/1 -> F 11.1Notify user (Logout Successful)/1(ResetConfirm)
  F 11.1Notify user (Logout Successful)/1(Logout Successful) -> Bus Element Out3/1
  F11.4 Provide User Interface/1(VisualsReady) -> F11.5 Recieve Credentials/1(VisualsReady)
  F11.5 Recieve Credentials/1(RecievedCredentials) -> F11.6 Verify Credentials/1(RecievedCredentials)
  F11.3 Recieve User Input/1(ReadytoInteract) -> F11.4 Provide User Interface/1(ReadytoInteract)
  F11.2 Turn ON System/1(WaitforInput) -> F11.3 Recieve User Input/1(WaitforInput)
  F11.8 Provide System Dashboard/1(DashboardLoaded) -> F11.10 Monitor System Parameters/2(DashboardLoaded)
  F11.6 Verify Credentials/1(Confirmation) -> F11.7 Confirm Login/1(Confirmation)
  Bus Element In4/1 -> F11.10 Monitor System Parameters/1(Stop Button)
  F11.7 Confirm Login/1(LOGINConfirm) -> Bus Element Out4/1
  Bus Element In5/1 -> F11.10 Monitor System Parameters/3(Faulty Product Detected)
  Bus Element In6/1 -> F11.10 Monitor System Parameters/5(Count)
  F11.15 Display System Parameters/1(SystemState) -> Bus Element Out5/1
  F11.15 Display System Parameters/2(LogoutPrompt) -> F11.14 Update Activity Log/1(LogoutPrompt)
  F11.15 Display System Parameters/3(observeparameters) -> F11.10 Monitor System Parameters/4(observeparameters)
  F11.10 Monitor System Parameters/1(NotifyEmergency) -> F11.11 Notify User/1(NotifyEmergency)
  F11.10 Monitor System Parameters/2(ShowParameters) -> F11.15 Display System Parameters/1(ShowParameters)
  Bus Element In7/1 -> F11.12Confirm System STOP/2(STOPConfirm)
  F11.14 Update Activity Log/1(LOGOUTConfirm) -> F11.12Confirm System STOP/1(LOGOUTConfirm)
  F11.14 Update Activity Log/2(DBUpdated) -> F11.13 Generate STOP Signal/1(DBUpdated)
  F11.12Confirm System STOP/1(Resetsystem) -> Bus Element Out6/1
  F11.13 Generate STOP Signal/1(STOPoperation) -> Bus Element Out2/1

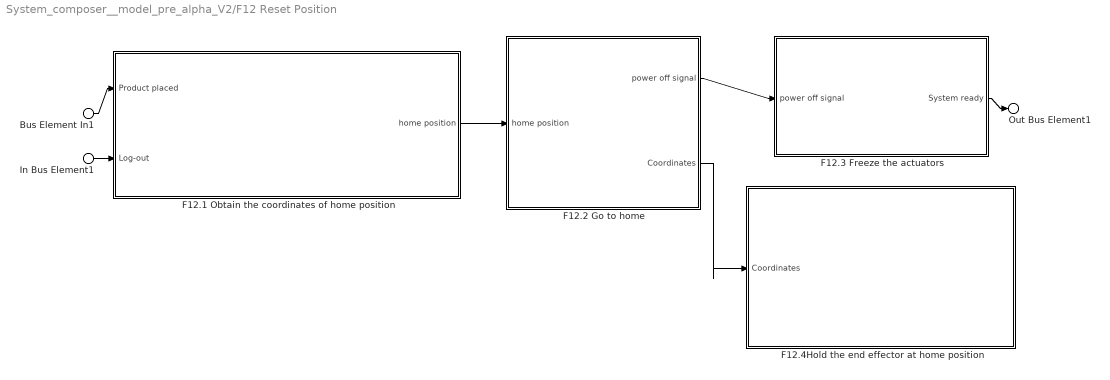
== system System_composer__model_pre_alpha_V2/F12 Reset Position ==
  Bus Element In1 : Inport  PortName=Product Placed
  In Bus Element1 : Inport  Port=2  PortName=Log-out
  F12.1 Obtain the coordinates of home position : Subsystem
      settings: PortSchema="{\"entries\":[{\"content\":{\"headerSize\":26,\"margin\":15,\"minimumSpacing\":25,\"sides\":[{\"content\":{\"connectorIds\":[\"In1\",\"In2\"]},\"type\":\"ConnectorPlacement.EquallySpacedRectSide\",\"uuid\":\"cfa9a458-ccb1-4b4b-9223-cdb6aaef5fc4\"},{\"content\":{\"connectorIds\":[\"Out1\"],\"side\":\"RIGHT\"},\"type\":\"ConnectorPlacement.EquallySpacedRectSide\",\"uuid\":\"f9e6f688-270f-46a5-8c07-32c6831cf3d3\"},{\"content\":{\"connectorIds\":[],\"side\":\"TOP\"},\"type\":\"ConnectorPlacement.EquallySpacedRectSide\",\"uuid\":\"2fcd258a-a10a-44a0-bcb2-682252ae81b0\"},{\"content\":{\"connectorIds\":[],\"side\":\"BOTTOM\"},\"type\":\"ConnectorPlacement.EquallySpacedRectSide\",\"uuid\":\"fd77c390-7ec2-4e40-9af2-fa45e616dbf4\"}]},\"type\":\"ConnectorPlacement.EquallySpacedConnector\",\"uuid\":\"80e45476-3fa2-42b9-aef1-d9f502108577\"}],\"packageUris\":[\"http://schema.mathworks.com/mf0/Connector/R2020b\"],\"version\":\"1.0\"}"
  F12.2 Go to home : Subsystem
      settings: PortSchema="{\"entries\":[{\"content\":{\"headerSize\":26,\"margin\":15,\"minimumSpacing\":25,\"sides\":[{\"content\":{\"connectorIds\":[\"In1\"]},\"type\":\"ConnectorPlacement.EquallySpacedRectSide\",\"uuid\":\"cfa9a458-ccb1-4b4b-9223-cdb6aaef5fc4\"},{\"content\":{\"connectorIds\":[\"Out2\",\"Out1\"],\"side\":\"RIGHT\"},\"type\":\"ConnectorPlacement.EquallySpacedRectSide\",\"uuid\":\"f9e6f688-270f-46a5-8c07-32c6831cf3d3\"},{\"content\":{\"connectorIds\":[],\"side\":\"TOP\"},\"type\":\"ConnectorPlacement.EquallySpacedRectSide\",\"uuid\":\"2fcd258a-a10a-44a0-bcb2-682252ae81b0\"}]},\"type\":\"ConnectorPlacement.EquallySpacedConnector\",\"uuid\":\"80e45476-3fa2-42b9-aef1-d9f502108577\"}],\"packageUris\":[\"http://schema.mathworks.com/mf0/Connector/R2020b\"],\"version\":\"1.0\"}"
  F12.3 Freeze the actuators : Subsystem
      settings: PortSchema="{\"entries\":[{\"content\":{\"headerSize\":26,\"margin\":15,\"minimumSpacing\":25,\"sides\":[{\"content\":{\"connectorIds\":[\"In1\"]},\"type\":\"ConnectorPlacement.EquallySpacedRectSide\",\"uuid\":\"cfa9a458-ccb1-4b4b-9223-cdb6aaef5fc4\"},{\"content\":{\"connectorIds\":[\"Out1\"],\"side\":\"RIGHT\"},\"type\":\"ConnectorPlacement.EquallySpacedRectSide\",\"uuid\":\"f9e6f688-270f-46a5-8c07-32c6831cf3d3\"},{\"content\":{\"connectorIds\":[],\"side\":\"TOP\"},\"type\":\"ConnectorPlacement.EquallySpacedRectSide\",\"uuid\":\"2fcd258a-a10a-44a0-bcb2-682252ae81b0\"}]},\"type\":\"ConnectorPlacement.EquallySpacedConnector\",\"uuid\":\"80e45476-3fa2-42b9-aef1-d9f502108577\"}],\"packageUris\":[\"http://schema.mathworks.com/mf0/Connector/R2020b\"],\"version\":\"1.0\"}"
  F12.4Hold the end effector at home position : Subsystem
      settings: PortSchema="{\"entries\":[{\"content\":{\"headerSize\":26,\"margin\":15,\"minimumSpacing\":25,\"sides\":[{\"content\":{\"connectorIds\":[\"In1\"]},\"type\":\"ConnectorPlacement.EquallySpacedRectSide\",\"uuid\":\"cfa9a458-ccb1-4b4b-9223-cdb6aaef5fc4\"},{\"content\":{\"connectorIds\":[],\"side\":\"RIGHT\"},\"type\":\"ConnectorPlacement.EquallySpacedRectSide\",\"uuid\":\"f9e6f688-270f-46a5-8c07-32c6831cf3d3\"},{\"content\":{\"connectorIds\":[],\"side\":\"TOP\"},\"type\":\"ConnectorPlacement.EquallySpacedRectSide\",\"uuid\":\"2fcd258a-a10a-44a0-bcb2-682252ae81b0\"}]},\"type\":\"ConnectorPlacement.EquallySpacedConnector\",\"uuid\":\"80e45476-3fa2-42b9-aef1-d9f502108577\"}],\"packageUris\":[\"http://schema.mathworks.com/mf0/Connector/R2020b\"],\"version\":\"1.0\"}"
  Out Bus Element1 : Outport  PortName=SystemReset
  wires:
  F12.3 Freeze the actuators/1(System ready) -> Out Bus Element1/1
  F12.2 Go to home/1(Coordinates) -> F12.4Hold the end effector at home position/1(Coordinates)
  F12.2 Go to home/2(power off signal) -> F12.3 Freeze the actuators/1(power off signal)
  In Bus Element1/1 -> F12.1 Obtain the coordinates of home position/2(Log-out)
  F12.1 Obtain the coordinates of home position/1(home position) -> F12.2 Go to home/1(home position)
  Bus Element In1/1 -> F12.1 Obtain the coordinates of home position/1(Product placed)

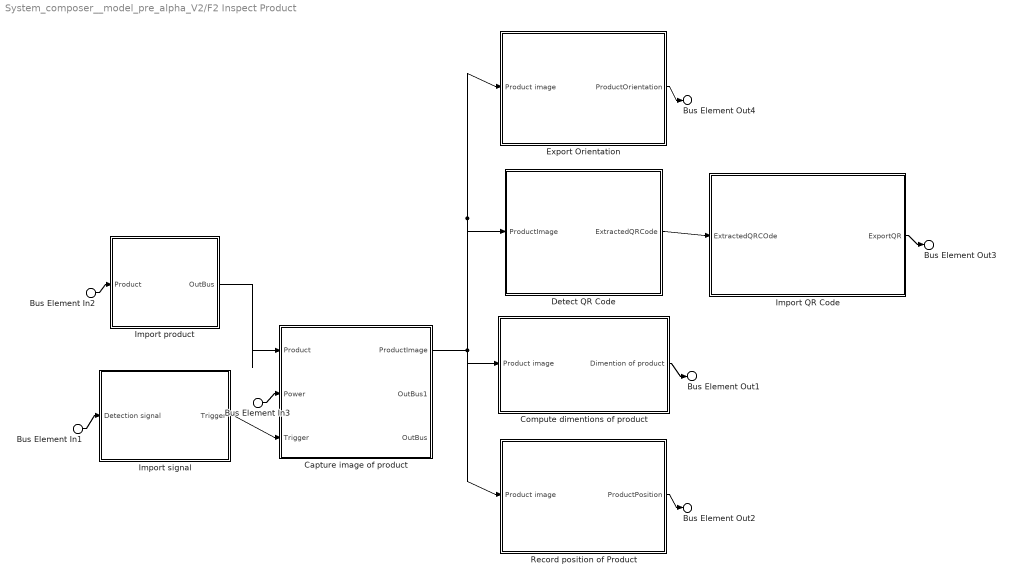
== system System_composer__model_pre_alpha_V2/F2 Inspect Product ==
  Bus Element In3 : Inport  PortName=Power
  Bus Element In2 : Inport  Port=2  PortName=Product
  Bus Element In1 : Inport  Port=3  PortName=Detection signal
  Capture image of product : Subsystem
      settings: PortSchema="{\"entries\":[{\"content\":{\"headerSize\":26,\"margin\":15,\"minimumSpacing\":25,\"sides\":[{\"content\":{\"connectorIds\":[\"In1\",\"In2\",\"In3\"]},\"type\":\"ConnectorPlacement.EquallySpacedRectSide\",\"uuid\":\"320e88d4-3d78-4d2f-ad02-b343723442c4\"},{\"content\":{\"connectorIds\":[\"Out1\",\"Out2\",\"Out3\"],\"side\":\"RIGHT\"},\"type\":\"ConnectorPlacement.EquallySpacedRectSide\",\"uuid\":\"09c33032-32ab-4ada-8ed8-0201f1b57dc0\"},{\"content\":{\"connectorIds\":[],\"side\":\"TOP\"},\"type\":\"ConnectorPlacement.EquallySpacedRectSide\",\"uuid\":\"2b028b26-f15f-43e2-ad75-04cde6dc5293\"}]},\"type\":\"ConnectorPlacement.EquallySpacedConnector\",\"uuid\":\"3dd2f29f-a920-492f-a094-d6d7756d0428\"}],\"packageUris\":[\"http://schema.mathworks.com/mf0/Connector/R2020b\"],\"version\":\"1.0\"}"
  Compute dimentions of product : Subsystem
      settings: PortSchema="{\"entries\":[{\"content\":{\"headerSize\":26,\"margin\":15,\"minimumSpacing\":25,\"sides\":[{\"content\":{\"connectorIds\":[\"In1\"]},\"type\":\"ConnectorPlacement.EquallySpacedRectSide\",\"uuid\":\"320e88d4-3d78-4d2f-ad02-b343723442c4\"},{\"content\":{\"connectorIds\":[\"Out1\"],\"side\":\"RIGHT\"},\"type\":\"ConnectorPlacement.EquallySpacedRectSide\",\"uuid\":\"09c33032-32ab-4ada-8ed8-0201f1b57dc0\"},{\"content\":{\"connectorIds\":[],\"side\":\"TOP\"},\"type\":\"ConnectorPlacement.EquallySpacedRectSide\",\"uuid\":\"2b028b26-f15f-43e2-ad75-04cde6dc5293\"}]},\"type\":\"ConnectorPlacement.EquallySpacedConnector\",\"uuid\":\"3dd2f29f-a920-492f-a094-d6d7756d0428\"}],\"packageUris\":[\"http://schema.mathworks.com/mf0/Connector/R2020b\"],\"version\":\"1.0\"}"
  Detect QR Code : Subsystem
      settings: PortSchema="{\"entries\":[{\"content\":{\"headerSize\":26,\"margin\":15,\"minimumSpacing\":25,\"sides\":[{\"content\":{\"connectorIds\":[\"In1\"]},\"type\":\"ConnectorPlacement.EquallySpacedRectSide\",\"uuid\":\"1c117138-a6d4-4ec0-b7b8-6d1428745998\"},{\"content\":{\"connectorIds\":[\"Out1\"],\"side\":\"RIGHT\"},\"type\":\"ConnectorPlacement.EquallySpacedRectSide\",\"uuid\":\"426d6ceb-18a6-42d8-9bd7-8fe69cb751f0\"},{\"content\":{\"connectorIds\":[],\"side\":\"TOP\"},\"type\":\"ConnectorPlacement.EquallySpacedRectSide\",\"uuid\":\"23012487-78cd-45b9-9306-44393710ac2e\"}]},\"type\":\"ConnectorPlacement.EquallySpacedConnector\",\"uuid\":\"f4468a7a-13e2-43af-b621-864ee5d109de\"}],\"packageUris\":[\"http://schema.mathworks.com/mf0/Connector/R2020b\"],\"version\":\"1.0\"}"
  Export Orientation : Subsystem
      settings: PortSchema="{\"entries\":[{\"content\":{\"headerSize\":26,\"margin\":15,\"minimumSpacing\":25,\"sides\":[{\"content\":{\"connectorIds\":[\"In1\"]},\"type\":\"ConnectorPlacement.EquallySpacedRectSide\",\"uuid\":\"320e88d4-3d78-4d2f-ad02-b343723442c4\"},{\"content\":{\"connectorIds\":[\"Out1\"],\"side\":\"RIGHT\"},\"type\":\"ConnectorPlacement.EquallySpacedRectSide\",\"uuid\":\"09c33032-32ab-4ada-8ed8-0201f1b57dc0\"},{\"content\":{\"connectorIds\":[],\"side\":\"TOP\"},\"type\":\"ConnectorPlacement.EquallySpacedRectSide\",\"uuid\":\"2b028b26-f15f-43e2-ad75-04cde6dc5293\"}]},\"type\":\"ConnectorPlacement.EquallySpacedConnector\",\"uuid\":\"3dd2f29f-a920-492f-a094-d6d7756d0428\"}],\"packageUris\":[\"http://schema.mathworks.com/mf0/Connector/R2020b\"],\"version\":\"1.0\"}"
  Import QR Code : Subsystem
      settings: PortSchema="{\"entries\":[{\"content\":{\"headerSize\":26,\"margin\":15,\"minimumSpacing\":25,\"sides\":[{\"content\":{\"connectorIds\":[\"In1\"]},\"type\":\"ConnectorPlacement.EquallySpacedRectSide\",\"uuid\":\"1c117138-a6d4-4ec0-b7b8-6d1428745998\"},{\"content\":{\"connectorIds\":[\"Out1\"],\"side\":\"RIGHT\"},\"type\":\"ConnectorPlacement.EquallySpacedRectSide\",\"uuid\":\"426d6ceb-18a6-42d8-9bd7-8fe69cb751f0\"},{\"content\":{\"connectorIds\":[],\"side\":\"TOP\"},\"type\":\"ConnectorPlacement.EquallySpacedRectSide\",\"uuid\":\"23012487-78cd-45b9-9306-44393710ac2e\"}]},\"type\":\"ConnectorPlacement.EquallySpacedConnector\",\"uuid\":\"f4468a7a-13e2-43af-b621-864ee5d109de\"}],\"packageUris\":[\"http://schema.mathworks.com/mf0/Connector/R2020b\"],\"version\":\"1.0\"}"
  Import product : Subsystem
      settings: PortSchema="{\"entries\":[{\"content\":{\"headerSize\":26,\"margin\":15,\"minimumSpacing\":25,\"sides\":[{\"content\":{\"connectorIds\":[\"In1\"]},\"type\":\"ConnectorPlacement.EquallySpacedRectSide\",\"uuid\":\"320e88d4-3d78-4d2f-ad02-b343723442c4\"},{\"content\":{\"connectorIds\":[\"Out1\"],\"side\":\"RIGHT\"},\"type\":\"ConnectorPlacement.EquallySpacedRectSide\",\"uuid\":\"09c33032-32ab-4ada-8ed8-0201f1b57dc0\"},{\"content\":{\"connectorIds\":[],\"side\":\"TOP\"},\"type\":\"ConnectorPlacement.EquallySpacedRectSide\",\"uuid\":\"2b028b26-f15f-43e2-ad75-04cde6dc5293\"}]},\"type\":\"ConnectorPlacement.EquallySpacedConnector\",\"uuid\":\"3dd2f29f-a920-492f-a094-d6d7756d0428\"}],\"packageUris\":[\"http://schema.mathworks.com/mf0/Connector/R2020b\"],\"version\":\"1.0\"}"
  Import signal : Subsystem
      settings: PortSchema="{\"entries\":[{\"content\":{\"headerSize\":26,\"margin\":15,\"minimumSpacing\":25,\"sides\":[{\"content\":{\"connectorIds\":[\"In1\"]},\"type\":\"ConnectorPlacement.EquallySpacedRectSide\",\"uuid\":\"320e88d4-3d78-4d2f-ad02-b343723442c4\"},{\"content\":{\"connectorIds\":[\"Out1\"],\"side\":\"RIGHT\"},\"type\":\"ConnectorPlacement.EquallySpacedRectSide\",\"uuid\":\"09c33032-32ab-4ada-8ed8-0201f1b57dc0\"},{\"content\":{\"connectorIds\":[],\"side\":\"TOP\"},\"type\":\"ConnectorPlacement.EquallySpacedRectSide\",\"uuid\":\"2b028b26-f15f-43e2-ad75-04cde6dc5293\"}]},\"type\":\"ConnectorPlacement.EquallySpacedConnector\",\"uuid\":\"3dd2f29f-a920-492f-a094-d6d7756d0428\"}],\"packageUris\":[\"http://schema.mathworks.com/mf0/Connector/R2020b\"],\"version\":\"1.0\"}"
  Record position of Product : Subsystem
      settings: PortSchema="{\"entries\":[{\"content\":{\"headerSize\":26,\"margin\":15,\"minimumSpacing\":25,\"sides\":[{\"content\":{\"connectorIds\":[\"In1\"]},\"type\":\"ConnectorPlacement.EquallySpacedRectSide\",\"uuid\":\"320e88d4-3d78-4d2f-ad02-b343723442c4\"},{\"content\":{\"connectorIds\":[\"Out1\"],\"side\":\"RIGHT\"},\"type\":\"ConnectorPlacement.EquallySpacedRectSide\",\"uuid\":\"09c33032-32ab-4ada-8ed8-0201f1b57dc0\"},{\"content\":{\"connectorIds\":[],\"side\":\"TOP\"},\"type\":\"ConnectorPlacement.EquallySpacedRectSide\",\"uuid\":\"2b028b26-f15f-43e2-ad75-04cde6dc5293\"}]},\"type\":\"ConnectorPlacement.EquallySpacedConnector\",\"uuid\":\"3dd2f29f-a920-492f-a094-d6d7756d0428\"}],\"packageUris\":[\"http://schema.mathworks.com/mf0/Connector/R2020b\"],\"version\":\"1.0\"}"
  Bus Element Out3 : Outport  PortName=ExportQR
  Bus Element Out1 : Outport  Port=2  PortName=Dimention of product
  Bus Element Out2 : Outport  Port=3  PortName=ProductPosition
  Bus Element Out4 : Outport  Port=4  PortName=ProductOrientation
  wires:
  Bus Element In3/1 -> Capture image of product/2(Power)
  Bus Element In1/1 -> Import signal/1(Detection signal)
  Bus Element In2/1 -> Import product/1(Product)
  Import product/1(OutBus) -> Capture image of product/1(Product)
  Capture image of product/1(ProductImage) -> Detect QR Code/1(ProductImage), Export Orientation/1(Product image), Compute dimentions of product/1(Product image), Record position of Product/1(Product image)
  Import signal/1(Trigger) -> Capture image of product/3(Trigger)
  Detect QR Code/1(ExtractedQRCode) -> Import QR Code/1(ExtractedQRCOde)
  Import QR Code/1(ExportQR) -> Bus Element Out3/1
  Export Orientation/1(ProductOrientation) -> Bus Element Out4/1
  Compute dimentions of product/1(Dimention of product) -> Bus Element Out1/1
  Record position of Product/1(ProductPosition) -> Bus Element Out2/1
